simulink model "CalebsModel"  (Simulink 7.7)
settings: Solver=ode45  StartTime=0.0  StopTime=10  RelTol=1e-3
values from neighbouring files (symbols this model uses):
  b_surf = 1e5    (= 100000)    [ControlDesign.m]
  ContactPoint = 0.023    [ControlDesign.m]
  K_backemf = 1000*mean( K_backemf_array )    [ControlDesign.m]
  K_L12_Force = 0.00229181    [ControlDesign.m]    (also in ControlDesignForceModeLinear.m = 2.29181)
  K_PWM = PWM_res/V_rail    (= 83.3333333333)    [ControlDesign.m]    (also in ControlDesignForceModeLinear.m = 0.012)
  k_surf = 1e8    (= 100000000)    [ControlDesign.m]
  kisa = (-(z_1 + z_2 + z_3)*Jphat + 3*Jphat - Ts*ba - (Ts^2)*ksa)/(Ts^3)    [ControlDesign.m]
  ksa = (-(z_1*z_2 + z_1*z_3 + z_2*z_3)*Jphat + 3*Jphat - 2*Ts*ba)/(Ts^2)    [ControlDesign.m]
  L12_Offset_I = 0.012995    [ControlDesign.m]    (also in ControlDesignForceModeLinear.m = 12.995)
  L_Range = [0 0.050]    [ControlDesign.m]    (also in ControlDesignForceModeLinear.m = [0 50]; VariableQpts.m = [0 50])
  m_surf = 1e3    (= 1000)    [ControlDesign.m]
  Mar = 0.075    [ControlDesign.m]    (also in ControlDesignForceModeLinear.m)
  PWM_res = 2000    [ControlDesign.m]    (also in ControlDesignForceModeLinear.m)
  Ra_L12 = 60    [ControlDesign.m]    (also in ControlDesignForceModeLinear.m)
  Ts = 1/fs    (= 0.001)    [ControlDesign.m]    (also in ControlDesignForceModeLinear.m)
undefined symbols (not defined in the file or in its folder): DiscIntNeverNeededParam
libraries: simulink x4
settings Model: Creator=secrest  LastModifiedBy=Caleb
settings DataIOCC: SignalLoggingSaveFormat=Dataset
settings OptimizationCC: ExpressionDepthLimit=128
settings DebuggingCC: UnderspecifiedInitializationDetection=Simplified  StateNameClashWarn=none
settings CodeAppCC: CustomSymbolStrType=$N$R$M_T
settings GRTTargetCC: TargetFunctionLibrary=NOT IN USE  CombineOutputUpdateFcns=on  CPPClassGenCompliant=on

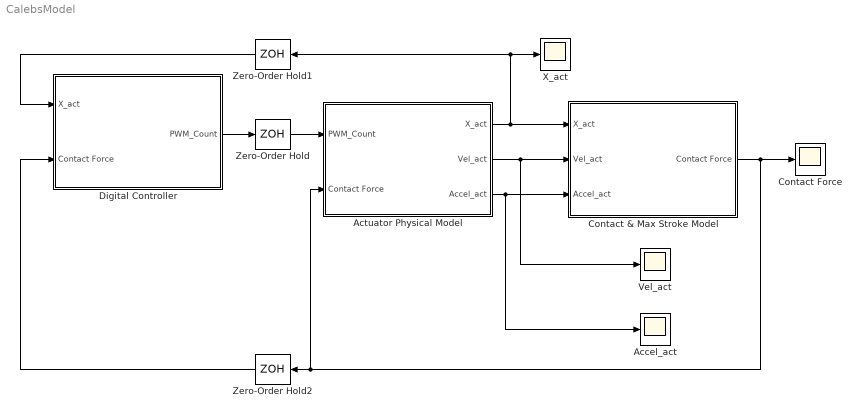
== system CalebsModel ==
  Accel_act : Scope
      settings: YMin=0  YMax=2300  SaveName=ScopeData3
  Actuator Physical Model : Subsystem
  Contact & Max Stroke Model : Subsystem
  Contact Force : Scope
      settings: YMin=-122.5  YMax=-116
  Digital Controller : Subsystem
  Vel_act : Scope
      settings: YMin=0  YMax=0.013  SaveName=ScopeData2
  X_act : Scope
      settings: YMin=0  YMax=0.017
  Zero-Order Hold : ZeroOrderHold  SampleTime=Ts
  Zero-Order Hold1 : ZeroOrderHold  SampleTime=Ts
  Zero-Order Hold2 : ZeroOrderHold  SampleTime=Ts
  wires:
  Actuator Physical Model/1(X_act) -> Contact & Max Stroke Model/1(X_act), X_act/1, Zero-Order Hold1/1
  Actuator Physical Model/2(Vel_act) -> Contact & Max Stroke Model/2(Vel_act), Vel_act/1
  Actuator Physical Model/3(Accel_act) -> Contact & Max Stroke Model/3(Accel_act), Accel_act/1
  Contact & Max Stroke Model/1(Contact Force) -> Contact Force/1, Actuator Physical Model/2(Contact Force), Zero-Order Hold2/1
  Digital Controller/1(PWM_Count) -> Zero-Order Hold/1
  Zero-Order Hold/1 -> Actuator Physical Model/1(PWM_Count)
  Zero-Order Hold1/1 -> Digital Controller/1(X_act)
  Zero-Order Hold2/1 -> Digital Controller/2(Contact Force)

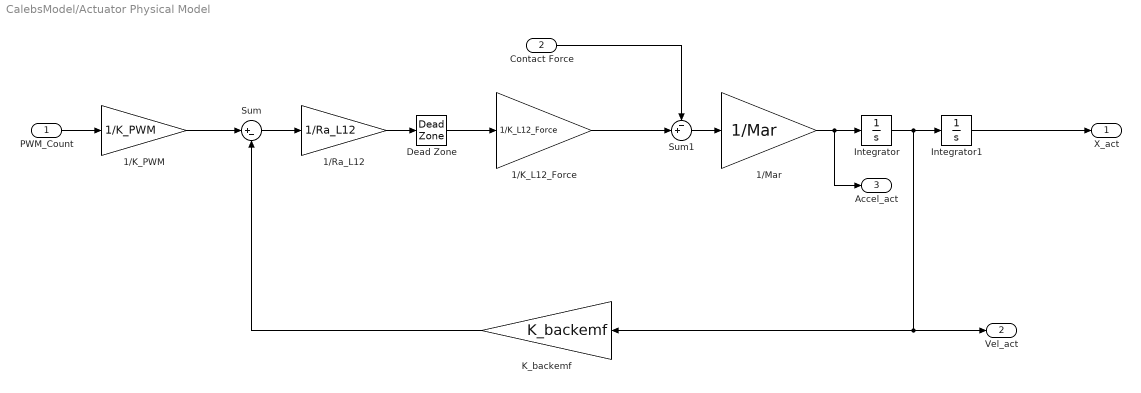
== system CalebsModel/Actuator Physical Model ==
  PWM_Count : Inport
  Contact Force : Inport  Port=2
  1/K_L12_Force : Gain  Gain=1/K_L12_Force
  1/K_PWM : Gain  Gain=1/K_PWM
  1/Mar : Gain  Gain=1/Mar
  1/Ra_L12 : Gain  Gain=1/Ra_L12
  Dead Zone : DeadZone  LowerValue=-L12_Offset_I  UpperValue=L12_Offset_I  SaturateOnIntegerOverflow=on
  Integrator : Integrator
  Integrator1 : Integrator
  K_backemf : Gain  Gain=K_backemf
  Sum : Sum  Inputs=|+-
  Sum1 : Sum  Inputs=-+|
  X_act : Outport
  Vel_act : Outport  Port=2
  Accel_act : Outport  Port=3
  wires:
  Sum1/1 -> 1/Mar/1
  1/Ra_L12/1 -> Dead Zone/1
  1/K_PWM/1 -> Sum/1
  Dead Zone/1 -> 1/K_L12_Force/1
  Sum/1 -> 1/Ra_L12/1
  K_backemf/1 -> Sum/2
  1/K_L12_Force/1 -> Sum1/2
  Integrator1/1 -> X_act/1
  Integrator/1 -> Integrator1/1, K_backemf/1, Vel_act/1
  Contact Force/1 -> Sum1/1
  1/Mar/1 -> Accel_act/1, Integrator/1
  PWM_Count/1 -> 1/K_PWM/1

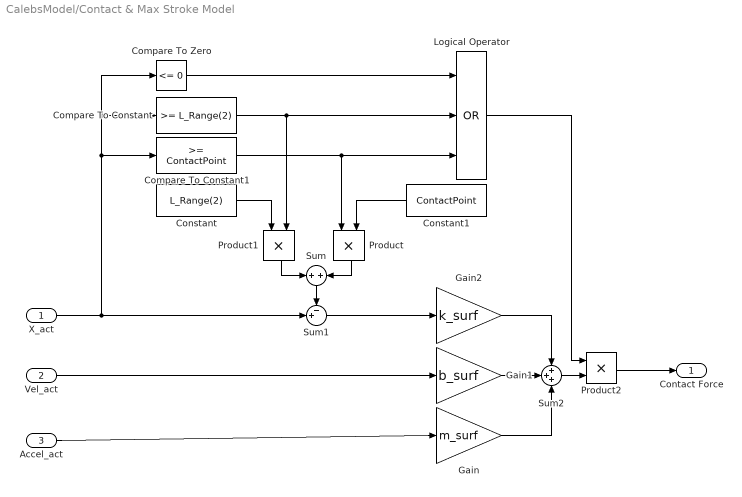
== system CalebsModel/Contact & Max Stroke Model ==
  X_act : Inport
  Vel_act : Inport  Port=2
  Accel_act : Inport  Port=3
  Compare To Constant : simulink/Logic and Bit Operations/Compare To Constant  SystemSampleTime=-1  relop=>=  const=L_Range(2)  LogicOutDataTypeMode=uint8
  Compare To Constant1 : simulink/Logic and Bit Operations/Compare To Constant  SystemSampleTime=-1  relop=>=  const=ContactPoint  LogicOutDataTypeMode=uint8
  Compare To Zero : simulink/Logic and Bit Operations/Compare To Zero  SystemSampleTime=-1  relop=<=  LogicOutDataTypeMode=uint8
  Constant : Constant  Value=L_Range(2)
  Constant1 : Constant  Value=ContactPoint
  Gain : Gain  Gain=m_surf
  Gain1 : Gain  Gain=b_surf
  Gain2 : Gain  Gain=k_surf
  Logical Operator : Logic  Operator=OR  Inputs=3  AllPortsSameDT=off  OutDataTypeStr=boolean
  Product : Product  RndMeth=Zero
  Product1 : Product  RndMeth=Zero
  Product2 : Product  RndMeth=Zero
  Sum : Sum  Inputs=+|+
  Sum1 : Sum  Inputs=-+|
  Sum2 : Sum  Inputs=+++
  Contact Force : Outport
  wires:
  X_act/1 -> Sum1/2, Compare To Zero/1, Compare To Constant/1, Compare To Constant1/1
  Compare To Zero/1 -> Logical Operator/1
  Vel_act/1 -> Gain1/1
  Accel_act/1 -> Gain/1
  Sum/1 -> Sum1/1
  Sum1/1 -> Gain2/1
  Constant/1 -> Product1/1
  Constant1/1 -> Product/2
  Gain2/1 -> Sum2/1
  Gain1/1 -> Sum2/2
  Gain/1 -> Sum2/3
  Logical Operator/1 -> Product2/1
  Sum2/1 -> Product2/2
  Product2/1 -> Contact Force/1
  Compare To Constant/1 -> Logical Operator/2, Product1/2
  Product1/1 -> Sum/1
  Compare To Constant1/1 -> Logical Operator/3, Product/1
  Product/1 -> Sum/2

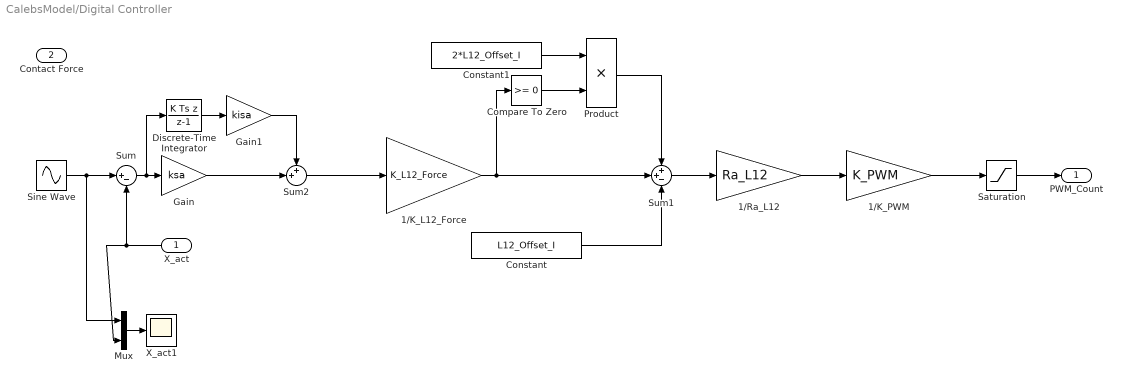
== system CalebsModel/Digital Controller ==
  X_act : Inport
  Contact Force : Inport  Port=2
  1/K_L12_Force : Gain  Gain=K_L12_Force
  1/K_PWM : Gain  Gain=K_PWM
  1/Ra_L12 : Gain  Gain=Ra_L12
  Compare To Zero : simulink/Logic and Bit Operations/Compare To Zero  SystemSampleTime=-1  relop=>=  LogicOutDataTypeMode=uint8
  Constant : Constant  Value=L12_Offset_I
  Constant1 : Constant  Value=2*L12_Offset_I
  Discrete-Time Integrator : DiscreteIntegrator  IntegratorMethod=Integration: Backward Euler  SampleTime=Ts  ICPrevOutput=DiscIntNeverNeededParam  ICPrevScaledInput=DiscIntNeverNeededParam
  Gain : Gain  Gain=ksa
  Gain1 : Gain  Gain=kisa
  Mux : Mux  Inputs=2
  Product : Product  RndMeth=Zero
  Saturation : Saturate  UpperLimit=PWM_res  LowerLimit=-PWM_res
  Sine Wave : Sin  Amplitude=0.005  Bias=0.01  Frequency=2*pi*0.25  SampleTime=Ts
  Sum : Sum  Inputs=|+-
  Sum1 : Sum  Inputs=++-
  Sum2 : Sum  Inputs=++|
  X_act1 : Scope
      settings: YMin=0  YMax=0.021  SaveName=ScopeData4
  PWM_Count : Outport
  wires:
  Sine Wave/1 -> Sum/1, Mux/1
  X_act/1 -> Sum/2, Mux/2
  Sum/1 -> Gain/1, Discrete-Time Integrator/1
  1/Ra_L12/1 -> 1/K_PWM/1
  1/K_PWM/1 -> Saturation/1
  1/K_L12_Force/1 -> Sum1/2, Compare To Zero/1
  Constant/1 -> Sum1/3
  Constant1/1 -> Product/1
  Compare To Zero/1 -> Product/2
  Product/1 -> Sum1/1
  Sum1/1 -> 1/Ra_L12/1
  Saturation/1 -> PWM_Count/1
  Discrete-Time Integrator/1 -> Gain1/1
  Gain1/1 -> Sum2/1
  Gain/1 -> Sum2/2
  Sum2/1 -> 1/K_L12_Force/1
  Mux/1 -> X_act1/1
